simulink model "ThreePhaseFullBridgeRec"  (R2021a)
settings: Solver=VariableStepAuto  StartTime=0.0  StopTime=0.1  RelTol=1e-3
libraries: spsVoltageMeasurementLib x6, spsDiodeLib x6, spsACVoltageSourceLib x3, spsCurrentMeasurementLib x2, spsSeriesRLCBranchLib x1, spsThreePhaseSeriesRLCBranchLib x1, spspowerguiLib x1
settings Model: Creator=EREN-PC  LastModifiedBy=EREN-PC
settings DataIOCC: ReturnWorkspaceOutputs=off

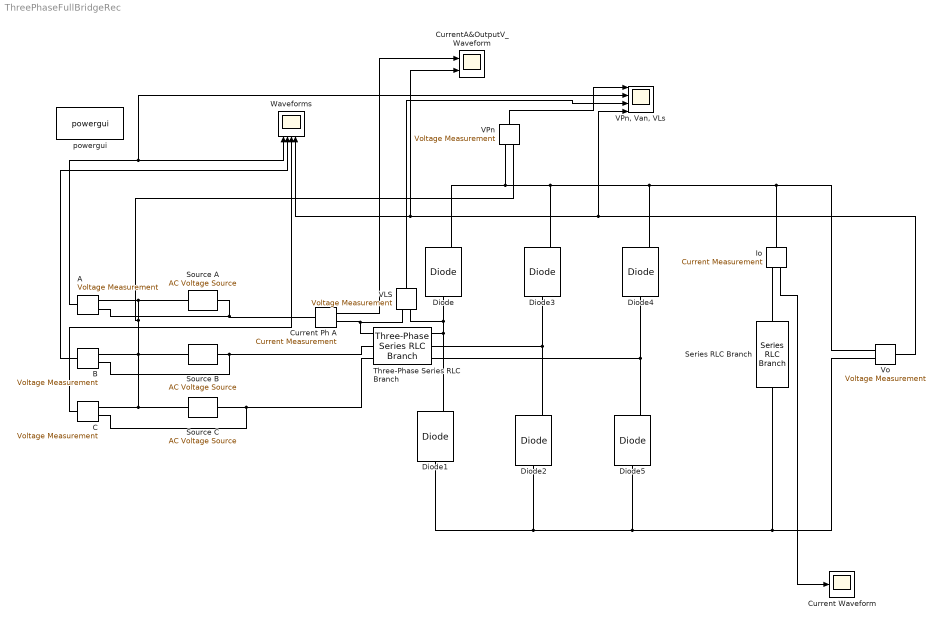
== system ThreePhaseFullBridgeRec ==
  A : spsVoltageMeasurementLib/Voltage Measurement  PhasorSimulation=off  OutputType=Complex  PSBequivalent=0
  B : spsVoltageMeasurementLib/Voltage Measurement  PhasorSimulation=off  OutputType=Complex  PSBequivalent=0
  C : spsVoltageMeasurementLib/Voltage Measurement  PhasorSimulation=off  OutputType=Complex  PSBequivalent=0
  Current Ph A : spsCurrentMeasurementLib/Current Measurement  PhasorSimulation=off  OutputType=Complex  PSBequivalent=0
  Current Waveform : Scope
  CurrentA&OutputV_Waveform : Scope  NumInputPorts=2
  Diode{,1..5} (6 alike) : spsDiodeLib/Diode  Ron=0.001  Lon=0  Vf=0.8  IC=0  UseSnubber=0  Rs=500  Cs=250e-9  Measurements=on
  Io : spsCurrentMeasurementLib/Current Measurement  PhasorSimulation=off  OutputType=Complex  PSBequivalent=0
  Series RLC Branch : spsSeriesRLCBranchLib/Series RLC Branch  LConnTagsString=__new0  RConnTagsString=__new0  BranchType=R  Resistance=10  Inductance=1e-3  SetiL0=off  InitialCurrent=0  Capacitance=1e-6  Setx0=off  InitialVoltage=0  Measurements=None
  Source A : spsACVoltageSourceLib/AC Voltage Source  Amplitude=320  Phase=0  Frequency=50  SampleTime=0  Measurements=None  BusType=swing  Pref=10e3  Qref=0  Qmin=-inf  Qmax=+inf
  Source B : spsACVoltageSourceLib/AC Voltage Source  Amplitude=320  Phase=120  Frequency=50  SampleTime=0  Measurements=None  BusType=swing  Pref=10e3  Qref=0  Qmin=-inf  Qmax=+inf
  Source C : spsACVoltageSourceLib/AC Voltage Source  Amplitude=320  Phase=240  Frequency=50  SampleTime=0  Measurements=None  BusType=swing  Pref=10e3  Qref=0  Qmin=-inf  Qmax=+inf
  Three-Phase Series RLC Branch : spsThreePhaseSeriesRLCBranchLib/Three-Phase Series RLC Branch  LConnTagsString=A|B|C  RConnTagsString=A|B|C  BranchType=L  Resistance=1  Inductance=10e-3  Capacitance=1e-6  Measurements=None
  VLS : spsVoltageMeasurementLib/Voltage Measurement  PhasorSimulation=off  OutputType=Complex  PSBequivalent=0
  VPn : spsVoltageMeasurementLib/Voltage Measurement  PhasorSimulation=off  OutputType=Complex  PSBequivalent=0
  "VPn, Van, VLs" : Scope  NumInputPorts=4
  Vo : spsVoltageMeasurementLib/Voltage Measurement  PhasorSimulation=off  OutputType=Complex  PSBequivalent=0
  Waveforms : Scope  NumInputPorts=5
  powergui : spspowerguiLib/powergui  Priority=1  SimulationMode=Discrete  SampleTime=1e-6  frequency=60  Iterations=50  frequencyindice=0  Pbase=100e6  ErrMax=1e-4  UnitsV=kV  UnitsW=MW  buscounter=0  FunctionMessages=off  echomessages=off  EnableUseOfTLC=off  CurrentSourceSwitches=off  DisableSnubberDevices=off  DisableRonSwitches=off  DisableVfSwitches=off  DisplayEquations=off  AutomaticDiscreteSolvers=off  SolverType=Tustin/Backward Euler (TBE)  Interpol=off  ExternalGateDelay=off  methode=off  Ts=100  x0status=blocks  SPID=on  SwTol=0  HookPort=off  NonlinearTolerance=1e-4  nMaxIteration=100  ContinueOnMaxIteration=off  RestoreLinks=warning  ResistiveCurrentMeasurement=off  Frange=[0:2:500]  Ylog=off  Xlog=on  ShowGrid=off  save=off  variable=ZData  structure=0  ZoomFFT=off  StartTime=0.0  cycles=1  DisplayStyle=1  fundamental=60  FreqAxis=off  MaxFrequency=1000  frequencyindicesteady=1  RmsSteady=1  display=off
  wires:
  Vo/1 -> "VPn, Van, VLs"/4, CurrentA&OutputV_Waveform/2, Waveforms/4
  A/1 -> "VPn, Van, VLs"/2, Waveforms/1
  B/1 -> Waveforms/2
  C/1 -> Waveforms/3
  Io/1 -> Current Waveform/1
  Current Ph A/1 -> CurrentA&OutputV_Waveform/1
  VPn/1 -> "VPn, Van, VLs"/1
  VLS/1 -> "VPn, Van, VLs"/3
  connections:
  B/LConn1 -- Three-Phase Series RLC Branch/LConn2 -- Source B/RConn1
  Diode1/RConn1 -- Three-Phase Series RLC Branch/RConn1 -- VLS/LConn2 -- Diode/LConn1
  Diode/RConn1 -- VPn/LConn1 -- Diode3/RConn1 -- Io/LConn1 -- Vo/LConn1 -- Diode4/RConn1
  Diode1/LConn1 -- Diode2/LConn1 -- Series RLC Branch/RConn1 -- Vo/LConn2 -- Diode5/LConn1
  Io/RConn1 -- Series RLC Branch/LConn1
  Diode5/RConn1 -- Diode4/LConn1 -- Three-Phase Series RLC Branch/RConn3
  Source A/LConn1 -- VPn/LConn2 -- B/LConn2 -- Source B/LConn1 -- C/LConn2 -- Source C/LConn1 -- A/LConn2
  A/LConn1 -- Source A/RConn1 -- Current Ph A/LConn1
  Diode2/RConn1 -- Three-Phase Series RLC Branch/RConn2 -- Diode3/LConn1
  C/LConn1 -- Source C/RConn1 -- Three-Phase Series RLC Branch/LConn3
  Three-Phase Series RLC Branch/LConn1 -- VLS/LConn1 -- Current Ph A/RConn1
